simulink model "bitirme0"  (R2023b)
settings: Solver=FixedStepAuto  StartTime=0.0  StopTime=45  RelTol=1e-3  EnableMultiTasking=on
libraries: stm32f4xxblockslib x11, stm32blockslib x4, simulink x1, lidarlib x1, slrealtimeiplib x1
settings Model: Creator=The MathWorks, Inc.  LastModifiedBy=yigit
settings OptimizationCC: EnhancedBackFolding=on  PassReuseOutputArgsAs=Individual arguments  ZeroExternalMemoryAtStartup=off  ZeroInternalMemoryAtStartup=off  MaxStackSize=64  OptimizeBlockOrder=speed  DifferentSizesBufferReuse=on  OptimizationCustomize=off  EfficientTunableParamExpr=on
settings DebuggingCC: ParameterTunabilityLossMsg=error  UnconnectedInputMsg=warning  UnconnectedOutputMsg=warning  UnconnectedLineMsg=warning  SubsystemReferenceDiagnosticForUnitTest=warning
settings HardwareCC: ProdBitPerPointer=32  ProdBitPerSizeT=32  ProdBitPerPtrDiffT=32  ProdLargestAtomicInteger=Long  ProdLargestAtomicFloat=Double  ProdWordSize=32  ProdLongLongMode=on  ProdHWDeviceType=ARM Compatible->ARM Cortex
settings ModelReferenceCC: EnableRefExpFcnMdlSchedulingChecks=on
settings SFSimCC: MATLABDynamicMemAlloc=off
settings RTWCC: Description=Embedded Coder  SystemTargetFile=ert.tlc  HardwareBoard=STM32F4xx Based  TemplateMakefile=ert_default_tmf  Toolchain=GNU Tools for ARM Embedded Processors  DLArmComputeVersion=19.05
settings CodeAppCC: ForceParamTrailComments=on  IgnoreCustomStorageClasses=off  OperatorAnnotations=on  SimulinkDataObjDesc=on  SFDataObjDesc=on  InsertBlockDesc=on
settings ERTTargetCC: CodeReplacementLibrary=ARM Cortex-M  ExtModeTransport=3  ExtModeStaticAlloc=on  ExtModeStaticAllocSize=8000  ExtModeMexFile=ext_xcp  ExtModeIntrfLevel=Level2 - Open

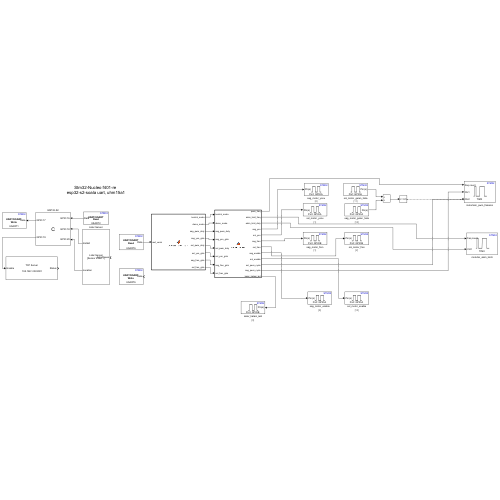
[thumbnail: Simulink's stored preview of the top-level diagram]
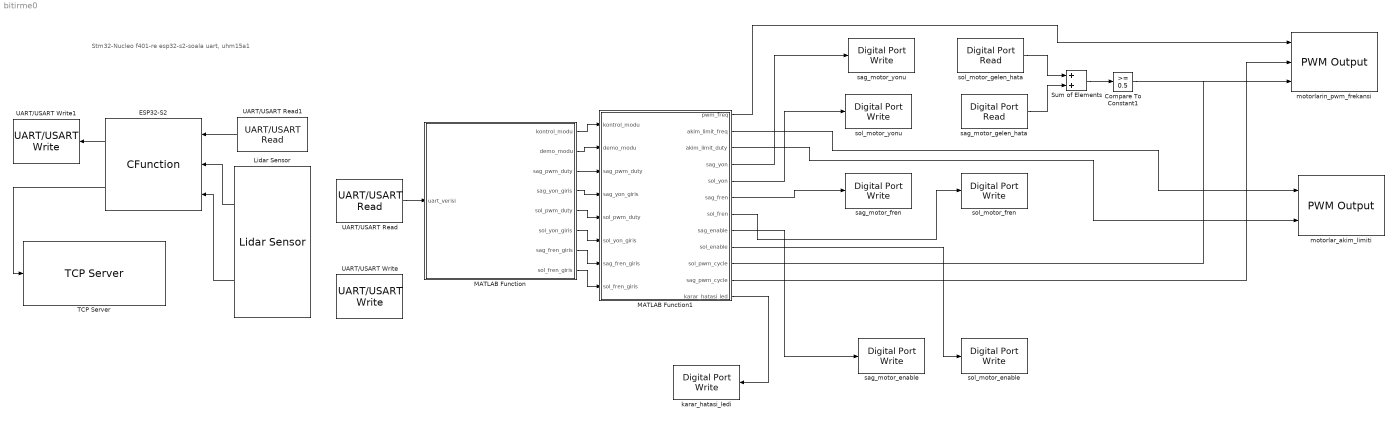
== system bitirme0 ==
  note: Stm32-Nucleo f401-re
      | esp32-s2-soala uart, uhm15a1
  Compare To Constant1 : simulink/Logic and Bit Operations/Compare To Constant  relop=>=  const=0.5  OutDataTypeStr=boolean
  ESP32-S2 : CFunction  StartCode=|
      | function [motor1_speed, motor2_speed, duration] = simulateESP32Block()
      | %#codegen
      | 
      | % Define the function to simulate ESP32 behavior
      | coder.inline('never');
      | coder.extrinsic('rand');
      | 
      | % Initialize the motor control data structure
      | data.motor1_speed = uint8(0);
      | data.motor2_speed = uint8(0);
      | data.duration = uint8(0);
      | 
      | % Call the function to simulate ESP32 behavior
      | data = simulateESP32();
      | 
      | % Extract the fields from the structure
      | motor1_speed = data.motor1_speed;
      | motor2_speed = data.motor2_speed;
      | duration = data.duration;
      | 
      | end
      | 
      | % Define the function simulateESP32 within the same file
      | function data = simulateESP32()
      | % Simulate receiving motor control data
      | 
      | % Initialize random seed
      | coder.extrinsic('rng');
      | rng('shuffle');
      | 
      | % Create a structure for motor control data
      | data.motor1_speed = uint8(rand() * 255);
      | data.motor2_speed = uint8(rand() * 255);
      | data.duration = uint8(rand() * 60);
      | 
      | end
  Lidar Sensor : lidarlib/Lidar Sensor  SensorIndex=1  UpdateRate=0.1  SensorPosition=[0 0.2 0]  SensorOrientation=[0 0 0]  ActorProfilesVariableName=disable  HostID=1  MaxRange=120  AzimuthLimits=[-180 180]  AzimuthResolution=0.16  UseCustomElevationAngles=off  ElevationAngles=[-25 -15.6 -11.3 -8.8:0.9:-4 -4:0.32:1.6 3.3 4.6 7 10.3 15]  ElevationLimits=[-20 20]  ElevationResolution=1.25  HasNoise=on  RangeAccuracy=0.002  FogVisibility=1000  Rainrate=0  OutputIntensity=off  OutputClusters=off
  MATLAB Function : MATLAB Function  TreatAsAtomicUnit=on
  MATLAB Function1 : MATLAB Function  TreatAsAtomicUnit=on
  Sum of Elements : Sum  OutMin=2
  TCP Server : slrealtimeiplib/TCP Server  Priority=-1  useHostTargetConn=off  serverAddress=192.168.1.95  serverPort=8001
  UART/USART Read : stm32blockslib/UART//USART Read  Priority=2  UARTModule=USART6  DataType=uint8  DataLength=8  BlockingMode=off  BlockingTimeout=0.1  OutputLength=off  OutputStatus=off  SampleTime=-1
      settings: LibrarySourceBlock=stm32f4xxblockslib/UART//USART Read
  UART/USART Read1 : stm32blockslib/UART//USART Read  Priority=2  UARTModule=USART2  DataType=uint8  DataLength=8  BlockingMode=off  BlockingTimeout=0.1  OutputLength=off  OutputStatus=off  SampleTime=-1
      settings: LibrarySourceBlock=stm32f4xxblockslib/UART//USART Read
  UART/USART Write : stm32blockslib/UART//USART Write  Priority=1  UARTModule=USART6  LengthOfDataToSend=off  BlockingMode=off  BlockingTimeout=0.1  OutputStatus=off
      settings: LibrarySourceBlock=stm32f4xxblockslib/UART//USART Write
  UART/USART Write1 : stm32blockslib/UART//USART Write  Priority=1  UARTModule=USART1  LengthOfDataToSend=off  BlockingMode=off  BlockingTimeout=0.1  OutputStatus=off
      settings: LibrarySourceBlock=stm32f4xxblockslib/UART//USART Write
  karar_hatasi_ledi : stm32f4xxblockslib/Digital Port Write  PortName=GPIOB  PinNumber=[0]  ReadOperation=off  IOAsArray=on  EnableSimPort=off
      settings: AttributesFormatString=%<PinNumber>
  motorlar_akim_limiti : stm32f4xxblockslib/PWM Output  TimerModule=TIM3  DutycycleUnits=Percentage  EnableChannel1=on  EnableChannel2=off  EnableChannel3=off  EnableChannel4=off  EnableCounterInput=off  EnableMainOutputInput=off  EnableFrequencyInput=on  SetRCAfterCE=off  OutputDirection=off  OutputMainOutputEnableStatus=off  SampleTime=0.1  EnableSimPort=off  EnableUpdateEvent=off  EnableCaptureCompare1Event=off  EnableCaptureCompare2Event=off  EnableCaptureCompare3Event=off  EnableCaptureCompare4Event=off  EnableTriggerEvent=off  EnableBreakEvent=on  ProcessorFamily=STM32F4  hoistedMaskSrc=ECSoC/ECSimCodegen/PWM Output
  motorlarin_pwm_frekansi : stm32f4xxblockslib/PWM Output  TimerModule=TIM3  DutycycleUnits=Percentage  EnableChannel1=on  EnableChannel2=on  EnableChannel3=off  EnableChannel4=off  EnableCounterInput=off  EnableMainOutputInput=off  EnableFrequencyInput=on  SetRCAfterCE=off  OutputDirection=off  OutputMainOutputEnableStatus=off  SampleTime=0.1  EnableSimPort=off  EnableUpdateEvent=off  EnableCaptureCompare1Event=off  EnableCaptureCompare2Event=off  EnableCaptureCompare3Event=off  EnableCaptureCompare4Event=off  EnableTriggerEvent=off  EnableBreakEvent=on  ProcessorFamily=STM32F4  hoistedMaskSrc=ECSoC/ECSimCodegen/PWM Output
  sag_motor_enable : stm32f4xxblockslib/Digital Port Write  PortName=GPIOA  PinNumber=[8]  ReadOperation=off  IOAsArray=on  EnableSimPort=off
      settings: AttributesFormatString=%<PinNumber>
  sag_motor_fren : stm32f4xxblockslib/Digital Port Write  PortName=GPIOB  PinNumber=[1]  ReadOperation=off  IOAsArray=on  EnableSimPort=off
      settings: AttributesFormatString=%<PinNumber>
  sag_motor_gelen_hata : stm32f4xxblockslib/Digital Port Read  PortName=GPIOA  PinNumber=[10]  ReadOperation=on  IOAsArray=on  SampleTime=-1  EnableSimPort=off
      settings: AttributesFormatString=%<PinNumber>
  sag_motor_yonu : stm32f4xxblockslib/Digital Port Write  PortName=GPIOA  PinNumber=[0]  ReadOperation=off  IOAsArray=on  EnableSimPort=off
      settings: AttributesFormatString=%<PinNumber>
  sol_motor_enable : stm32f4xxblockslib/Digital Port Write  PortName=GPIOA  PinNumber=[10]  ReadOperation=off  IOAsArray=on  EnableSimPort=off
      settings: AttributesFormatString=%<PinNumber>
  sol_motor_fren : stm32f4xxblockslib/Digital Port Write  PortName=GPIOB  PinNumber=[2]  ReadOperation=off  IOAsArray=on  EnableSimPort=off
      settings: AttributesFormatString=%<PinNumber>
  sol_motor_gelen_hata : stm32f4xxblockslib/Digital Port Read  PortName=GPIOA  PinNumber=[11]  ReadOperation=on  IOAsArray=on  SampleTime=-1  EnableSimPort=off
      settings: AttributesFormatString=%<PinNumber>
  sol_motor_yonu : stm32f4xxblockslib/Digital Port Write  PortName=GPIOA  PinNumber=[1]  ReadOperation=off  IOAsArray=on  EnableSimPort=off
      settings: AttributesFormatString=%<PinNumber>
  wires:
  UART/USART Read/1 -> MATLAB Function/1(uart_verisi)
  UART/USART Read1/1 -> ESP32-S2/1
  ESP32-S2/1 -> UART/USART Write1/1
  ESP32-S2/2 -> TCP Server/1
  Lidar Sensor/1 -> ESP32-S2/2
  Lidar Sensor/2 -> ESP32-S2/3
  MATLAB Function/1(kontrol_modu) -> MATLAB Function1/1(kontrol_modu)
  MATLAB Function/2(demo_modu) -> MATLAB Function1/2(demo_modu)
  MATLAB Function/3(sag_pwm_duty) -> MATLAB Function1/3(sag_pwm_duty)
  MATLAB Function/4(sag_yon_giris) -> MATLAB Function1/4(sag_yon_giris)
  MATLAB Function/6(sol_yon_giris) -> MATLAB Function1/6(sol_yon_giris)
  MATLAB Function/7(sag_fren_giris) -> MATLAB Function1/7(sag_fren_giris)
  MATLAB Function/8(sol_fren_giris) -> MATLAB Function1/8(sol_fren_giris)
  MATLAB Function/5(sol_pwm_duty) -> MATLAB Function1/5(sol_pwm_duty)
  MATLAB Function1/4(sag_yon) -> sag_motor_yonu/1
  Sum of Elements/1 -> Compare To Constant1/1
  Compare To Constant1/1 -> ?
  MATLAB Function1/5(sol_yon) -> sol_motor_yonu/1
  MATLAB Function1/7(sol_fren) -> sol_motor_fren/1
  MATLAB Function1/6(sag_fren) -> sag_motor_fren/1
  MATLAB Function1/12(karar_hatasi_led) -> karar_hatasi_ledi/1
  MATLAB Function1/8(sag_enable) -> sag_motor_enable/1
  MATLAB Function1/9(sol_enable) -> sol_motor_enable/1
  sol_motor_gelen_hata/1 -> Sum of Elements/1
  sag_motor_gelen_hata/1 -> Sum of Elements/2
  MATLAB Function1/1(pwm_freq) -> motorlarin_pwm_frekansi/1
  MATLAB Function1/11(sag_pwm_cycle) -> motorlarin_pwm_frekansi/2
  MATLAB Function1/10(sol_pwm_cycle) -> motorlarin_pwm_frekansi/3
  MATLAB Function1/2(akim_limit_freq) -> motorlar_akim_limiti/1
  MATLAB Function1/3(akim_limit_duty) -> motorlar_akim_limiti/2

== matlab function bitirme0/MATLAB Function1 ==
  data: pwm_freq output; akim_limit_freq output; akim_limit_duty output; sag_yon output; sol_yon output; sag_fren output; sol_fren output; sag_enable output; sol_enable output; sol_pwm_cycle output; kontrol_modu input; sag_pwm_cycle output; demo_modu input; sag_pwm_duty input; sag_yon_giris input; sol_pwm_duty input; sol_yon_giris input; sag_fren_giris input; sol_fren_giris input; karar_hatasi_led output
function [pwm_freq, akim_limit_freq, akim_limit_duty, sag_yon, sol_yon, sag_fren, sol_fren, sag_enable, sol_enable, sol_pwm_cycle, sag_pwm_cycle, karar_hatasi_led] = motor_secici(kontrol_modu, demo_modu, sag_pwm_duty, sag_yon_giris, sol_pwm_duty, sol_yon_giris, sag_fren_giris, sol_fren_giris)
%#codegen

% Sabit PWM frekansı
pwm_freq = 13.5e3;  % 13.5 kHz
akim_limit_freq = 20e3; % 20 kHz
akim_limit_duty = 0.7;  

% Başlangıç değerlerini ayarla
sag_pwm_cycle = 0.0;  % Sağ motor PWM duty cycle (0.0 to 1.0)
sag_yon = uint8(0);   % Sağ motor yön kontrolü
sol_pwm_cycle = 0.0;  % Sol motor PWM duty cycle (0.0 to 1.0)
sol_yon = uint8(0);   % Sol motor yön kontrolü
sag_enable = uint8(0);  % Sağ motor enable sinyali
sol_enable = uint8(0);  % Sol motor enable sinyali
sag_fren = uint8(0);   % Sağ motor fren sinyali
sol_fren = uint8(0);   % Sol motor fren sinyali
karar_hatasi_led = uint8(0); % Karar hatası LED

switch kontrol_modu
    case 1  % Manuel Kontrol
        if sag_pwm_duty > 0 || sag_yon_giris ~= 0
            % Sağ motor kontrol
            sag_enable = uint8(1);
            sag_pwm_cycle = sag_pwm_duty;
            sag_yon = sag_yon_giris;
        end
        if sol_pwm_duty > 0 || sol_yon_giris ~= 0
            % Sol motor kontrol
            sol_enable = uint8(1);
            sol_pwm_cycle = sol_pwm_duty;
            sol_yon = sol_yon_giris;
        end
        % Fren sinyalleri
        sag_fren = sag_fren_giris;
        sol_fren = sol_fren_giris;
        
    case 2  % Demo Modu
        if demo_modu == 1
            % Predefined sequence for demo mode
            sag_enable = uint8(1);
            sol_enable = uint8(1);
            sag_pwm_cycle = 1.0; % %100 duty cycle
            sol_pwm_cycle = 1.0; % %100 duty cycle
            pause(1);
            sag_pwm_cycle = 0.5; % %50 duty cycle
            sol_pwm_cycle = 0.5; % %50 duty cycle
            pause(1);
            sag_pwm_cycle = 0.8; % %80 duty cycle
            sol_pwm_cycle = 0.2; % %20 duty cycle
            pause(1);
            sag_pwm_cycle = 0.2; % %20 duty cycle
            sol_pwm_cycle = 0.8; % %80 duty cycle
            pause(1);
        else
            sag_enable = uint8(0);
            sol_enable = uint8(0);
        end
        
    case 3  % Fren
        sag_enable = uint8(0);
        sol_enable = uint8(0);
        sag_fren = sag_fren_giris;
        sol_fren = sol_fren_giris;
        
    otherwise  % Error state
        karar_hatasi_led = uint8(1);
        sag_enable = uint8(0);
        sol_enable = uint8(0);
        sag_pwm_cycle = 0.0;
        sag_yon = uint8(0);
        sol_pwm_cycle = 0.0;
        sol_yon = uint8(0);
        sag_fren = uint8(0);
        sol_fren = uint8(0);
end
end

== matlab function bitirme0/MATLAB Function ==
  data: uart_verisi input; kontrol_modu output; demo_modu output; sag_pwm_duty output; sag_yon_giris output; sol_pwm_duty output; sol_yon_giris output; sag_fren_giris output; sol_fren_giris output
function [kontrol_modu, demo_modu, sag_pwm_duty, sag_yon_giris, sol_pwm_duty, sol_yon_giris, sag_fren_giris, sol_fren_giris] = process_uart_data(uart_verisi)
    % UART verisini işleyerek kontrol sinyallerini çıkartır
    % Başlık çıkarma
    baslik = uart_verisi(1);
    
    % Varsayılan değerler
    kontrol_modu = uint8(2); % Başlangıç değeri olarak demo modu
    demo_modu = uint8(1); % Demo modu 1 seçeneği başlangıç olarak
    sag_pwm_duty = 0.0; % PWM duty cycle başlangıç olarak 0.0
    sag_yon_giris = uint8(0);
    sol_pwm_duty = 0.0; % PWM duty cycle başlangıç olarak 0.0
    sol_yon_giris = uint8(0);
    sag_fren_giris = uint8(0);
    sol_fren_giris = uint8(0);
    
    if baslik ~= 0xAA
        % Geçersiz başlık, varsayılan demo modu 1'i seç
        return;
    end
    
    % Kontrol modu, demo modu ve veriyi çıkarma
    kontrol_modu = uart_verisi(2);
    demo_modu = uart_verisi(3);
    kontrol_verisi = uart_verisi(4:7);  % Gerekli veri uzunluğuna göre ayarlandı
    fren_verisi = uart_verisi(8:9);     % Gerekli veri uzunluğuna göre ayarlandı
    
    % Kontrol verilerini değişkenlere atama
    sag_pwm_duty = double(kontrol_verisi(1)) / 255.0; % 0-255 arası değeri 0.0-1.0 arasına çevir
    sag_yon_giris = kontrol_verisi(2);
    sol_pwm_duty = double(kontrol_verisi(3)) / 255.0; % 0-255 arası değeri 0.0-1.0 arasına çevir
    sol_yon_giris = kontrol_verisi(4);
    sag_fren_giris = fren_verisi(1);
    sol_fren_giris = fren_verisi(2);
end
